simulink model "Scenario2"  (R2023a)
settings: Solver=VariableStepAuto  StartTime=0.0  StopTime=30  RelTol=1e-3
libraries: SignalEditorBlockLib x1
settings Model: Creator=Νίκος  LastModifiedBy=Νίκος

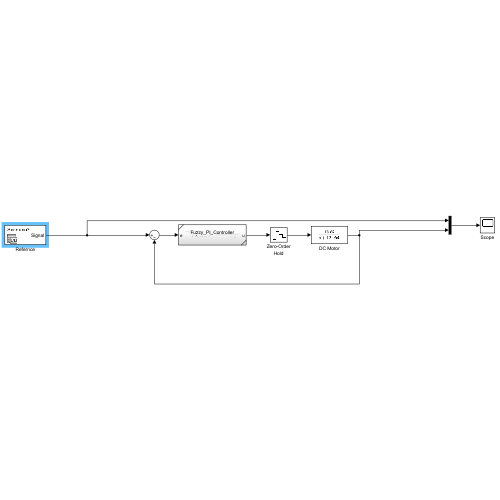
[thumbnail: Simulink's stored preview of the top-level diagram]
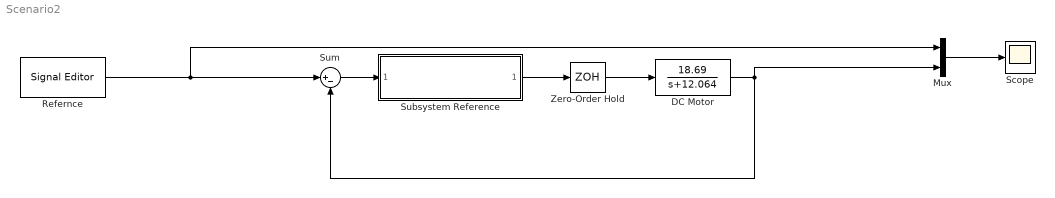
== system Scenario2 ==
  DC Motor : TransferFcn  Numerator=[18.69]  Denominator=[1 12.064]
  Mux : Mux  Inputs=2
  Refernce : SignalEditorBlockLib/Signal Editor  FileName=scenario2_input.mat  ActiveScenario=Scenario2  ActiveSignal=Signal  IsBus=off  OutputBusObjectStr=Bus: BusObject  SampleTime=0.01  ZeroCross=off  OutputAfterFinalValue=Setting to zero  Unit=inherit  PreserveSignalName=on  ApplySigPropsToAllScenarios=on
  Scope : Scope
  Subsystem Reference : Subsystem  ReferencedSubsystem=Fuzzy_PI_Controller
  Sum : Sum  Inputs=|+-
  Zero-Order Hold : ZeroOrderHold  SampleTime=-1
  wires:
  Refernce/1 -> Mux/1, Sum/1
  DC Motor/1 -> Mux/2, Sum/2
  Sum/1 -> Subsystem Reference/1
  Zero-Order Hold/1 -> DC Motor/1
  Mux/1 -> Scope/1
  Subsystem Reference/1 -> Zero-Order Hold/1
